simulink model "Practica3_ValeriaSinaiLaraRojas"  (R2025b)
settings: Solver=ode23t  StartTime=0.0  StopTime=10  RelTol=1e-3
libraries: fl_lib x22, nesl_utility x10
settings Model: Creator=Cecilia  LastModifiedBy=Cecilia

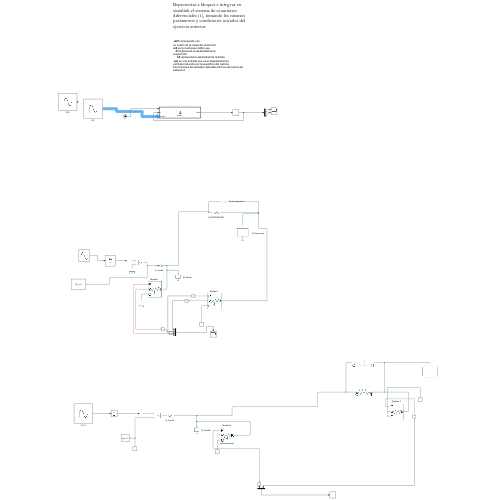
[thumbnail: Simulink's stored preview of the top-level diagram]
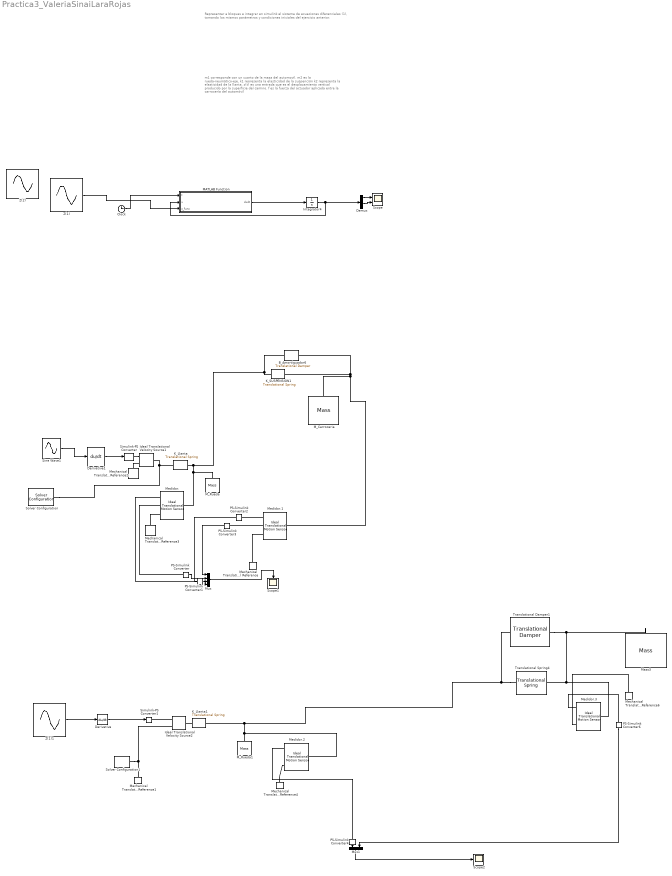
== system Practica3_ValeriaSinaiLaraRojas ==
  note: m1 corresponde con
      | un cuarto de la masa del automovil.
      | m2 es la rueda-neumático-eje,
      | k1 representa la elasticidad de la
      | suspención
      | k2 representa la elasticidad de la llanta.
      | z(t) es una entrada que es el desplazamiento
      | vertical producido por la superficie del camino.
      | f es la fuerza del actuador aplicada entre la carrocería del
      | automóvil
  note: Representar a bloques e integrar en simulink el sistema de ecuaciones diferenciales (1), tomando los mismos
      | parámetros y condiciones iniciales del ejercicio anterior.
  B_Amortiguador6 : fl_lib/Mechanical/Translational Elements/Translational Damper  D=1000 N*s/m  v_specify=off  v_priority=None  v=0 m/s  v_nominal_specify=off  v_nominal_value=1  v_nominal_unit=m/s  f_specify=off  f_priority=None  f=0 N  f_nominal_specify=off  f_nominal_value=1  f_nominal_unit=N
  Clock : Clock
  Demux : Demux
  Derivative : Derivative
  Derivative1 : Derivative
  Ideal Translational Velocity Source1 : fl_lib/Mechanical/Mechanical Sources/Ideal Translational Velocity Source
  Ideal Translational Velocity Source2 : fl_lib/Mechanical/Mechanical Sources/Ideal Translational Velocity Source
  Integrator4 : Integrator  InitialCondition=[0; 0; 0; 0]
  K_Llanta : fl_lib/Mechanical/Translational Elements/Translational Spring  spr_rate=19000 N/m  v_specify=off  v_priority=None  v=0 m/s  v_nominal_specify=off  v_nominal_value=1  v_nominal_unit=m/s  f_specify=off  f_priority=None  f=0 N  f_nominal_specify=off  f_nominal_value=1  f_nominal_unit=N  x_specify=off  x_priority=High  x=0 m  x_nominal_specify=off  x_nominal_value=1  x_nominal_unit=m
  K_Llanta1 : fl_lib/Mechanical/Translational Elements/Translational Spring  spr_rate=19000 N/m  v_specify=off  v_priority=None  v=0 m/s  v_nominal_specify=off  v_nominal_value=1  v_nominal_unit=m/s  f_specify=off  f_priority=None  f=0 N  f_nominal_specify=off  f_nominal_value=1  f_nominal_unit=N  x_specify=off  x_priority=High  x=0 m  x_nominal_specify=off  x_nominal_value=1  x_nominal_unit=m
  K_SUSPENSION1 : fl_lib/Mechanical/Translational Elements/Translational Spring  spr_rate=16182 N/m  v_specify=off  v_priority=None  v=0 m/s  v_nominal_specify=off  v_nominal_value=1  v_nominal_unit=m/s  f_specify=off  f_priority=None  f=0 N  f_nominal_specify=off  f_nominal_value=1  f_nominal_unit=N  x_specify=off  x_priority=High  x=0 m  x_nominal_specify=off  x_nominal_value=1  x_nominal_unit=m
  MATLAB Function : MATLAB Function  TreatAsAtomicUnit=on
  M_Carroceria : fl_lib/Mechanical/Translational Elements/Mass  mass=290 kg  num_ports=foundation.enum.numPorts2.one  v_specify=on  v_priority=High  v=1 m/s  v_nominal_specify=on  v_nominal_value=1  v_nominal_unit=m/s  f_specify=off  f_priority=None  f=0 N  f_nominal_specify=off  f_nominal_value=1  f_nominal_unit=N
  M_Rueda : fl_lib/Mechanical/Translational Elements/Mass  mass=59 kg  num_ports=foundation.enum.numPorts2.one  v_specify=off  v_priority=High  v=0 m/s  v_nominal_specify=off  v_nominal_value=1  v_nominal_unit=m/s  f_specify=off  f_priority=None  f=0 N  f_nominal_specify=off  f_nominal_value=1  f_nominal_unit=N
  M_Rueda1 : fl_lib/Mechanical/Translational Elements/Mass  mass=59 kg  num_ports=foundation.enum.numPorts2.one  v_specify=off  v_priority=High  v=0 m/s  v_nominal_specify=off  v_nominal_value=1  v_nominal_unit=m/s  f_specify=off  f_priority=None  f=0 N  f_nominal_specify=off  f_nominal_value=1  f_nominal_unit=N
  Mass3 : fl_lib/Mechanical/Translational Elements/Mass  mass=290 kg  num_ports=foundation.enum.numPorts2.one  v_specify=on  v_priority=High  v=0 m/s  v_nominal_specify=on  v_nominal_value=1  v_nominal_unit=m/s  f_specify=off  f_priority=None  f=0 N  f_nominal_specify=off  f_nominal_value=1  f_nominal_unit=N
  Mechanical Translational Reference{,1..4,6} (6 alike) : fl_lib/Mechanical/Translational Elements/Mechanical Translational Reference
  Medidor.{,1..3} (4 alike) : fl_lib/Mechanical/Mechanical Sensors/Ideal Translational Motion Sensor  reference=foundation.enum.MeasurementReference.difference  acceleration_port=false  velocity_port=true  position_port=true  offset=0 m
  Mux : Mux
  Mux1 : Mux  Inputs=2
  PS-Simulink Converter{,1..4,6} (6 alike) : nesl_utility/PS-Simulink Converter  PhysicalDomain=network_engine_domain  SubClassName=ps_output  LeftPortType=input  RightPortType=output  PseudoPeriodic=off  Frequencies=[]  VectorFormat=inherit  Unit=inherit  AffineConversion=off
  Scope : Scope  NumInputPorts=2
      settings: ActiveDisplayYMinimum=-0.061836360748085892  ActiveDisplayYMaximum=0.068675886807107581
  Scope1 : Scope
      settings: ActiveDisplayYMinimum=-1.0241021314644039  ActiveDisplayYMaximum=1.2249002368293782
  Scope2 : Scope
      settings: ActiveDisplayYMinimum=-0.12212269763999509  ActiveDisplayYMaximum=0.10067538321812189  DataLoggingVariableName=ScopeData2
  Simulink-PS Converter : nesl_utility/Simulink-PS Converter  PhysicalDomain=network_engine_domain  SubClassName=ps_input  LeftPortType=input  RightPortType=output  PseudoPeriodic=off  Frequencies=[]  NoiseDistribution=none  NoiseParameters=[]  Unit=1  AffineConversion=off  FilteringAndDerivatives=provide  SimscapeFilterOrder=1  InputFilterTimeConstant=0.001  UdotUserProvided=0
  Simulink-PS Converter1 : nesl_utility/Simulink-PS Converter  PhysicalDomain=network_engine_domain  SubClassName=ps_input  LeftPortType=input  RightPortType=output  PseudoPeriodic=off  Frequencies=[]  NoiseDistribution=none  NoiseParameters=[]  Unit=1  AffineConversion=off  FilteringAndDerivatives=provide  SimscapeFilterOrder=1  InputFilterTimeConstant=0.001  UdotUserProvided=0
  Sine Wave1 : Sin  Amplitude=0.05  Frequency=20*pi  SampleTime=0
  Solver Configuration : nesl_utility/Solver Configuration  PhysicalDomain=network_engine_domain  SubClassName=solver  LeftPortType=input  RightPortType=generic  Tones=[]  Harmonics=[]  SimulateNoise=off  Profile=off  UseLocalSampling=off  EnableSwitchedLinearOptims=on  FrequencyDomain=off  UseCCode=off  RelTol=0.001  AbsTol=0.001  MinStep=1e-09  ToWorkspace=off  RevertToSquareIcSolve=off  NumHomotopyIterations=100  PhasorMode=off  PhasorModeNumHarmonics=1  ConsistencySolver=NEWTON_XTOL_AFTER_FTOL  IndexReductionMethod=DerivativeReplacement  DoDC=off  ResidualTolerance=1e-09  ConsistencyTolSource=GLOBAL  ConsistencyAbsTol=0.001  ConsistencyRelTol=0.001  ConsistencyTolFactor=0.001  UseLocalSolver=off  LocalSolverChoice=NE_BACKWARD_EULER_ADVANCER  ResolveIndetEquations=on  FunctionEvalNumThread=1  LocalSolverSampleTime=0.001  DoFixedCost=off  MaxNonlinIter=3  MaxModeIter=2  ComputeImpulses=off  ImpulseIterations=2  LinearAlgebra=auto  LinearAlgebraNumThread=0  EquationFormulation=NE_TIME_EF  DelaysMemoryBudget=1024  AutomaticFiltering=on  FilteringTimeConstant=0.001  PartitionStorageMethod=AS_NEEDED  PartitionMemoryBudget=1024  PartitionMethod=ROBUST  MultibodyUseLocalSolver=off  MultibodyLocalSolverChoice=ODE1  MultibodyLocalSolverSampleTime=0.001
  Solver Configuration1 : nesl_utility/Solver Configuration  PhysicalDomain=network_engine_domain  SubClassName=solver  LeftPortType=input  RightPortType=generic  Tones=[]  Harmonics=[]  SimulateNoise=off  Profile=off  UseLocalSampling=off  EnableSwitchedLinearOptims=on  FrequencyDomain=off  UseCCode=off  RelTol=0.001  AbsTol=0.001  MinStep=1e-09  ToWorkspace=off  RevertToSquareIcSolve=off  NumHomotopyIterations=100  PhasorMode=off  PhasorModeNumHarmonics=1  ConsistencySolver=NEWTON_XTOL_AFTER_FTOL  IndexReductionMethod=DerivativeReplacement  DoDC=off  ResidualTolerance=1e-09  ConsistencyTolSource=GLOBAL  ConsistencyAbsTol=0.001  ConsistencyRelTol=0.001  ConsistencyTolFactor=0.001  UseLocalSolver=off  LocalSolverChoice=NE_BACKWARD_EULER_ADVANCER  ResolveIndetEquations=on  FunctionEvalNumThread=1  LocalSolverSampleTime=0.001  DoFixedCost=off  MaxNonlinIter=3  MaxModeIter=2  ComputeImpulses=off  ImpulseIterations=2  LinearAlgebra=auto  LinearAlgebraNumThread=0  EquationFormulation=NE_TIME_EF  DelaysMemoryBudget=1024  AutomaticFiltering=on  FilteringTimeConstant=0.001  PartitionStorageMethod=AS_NEEDED  PartitionMemoryBudget=1024  PartitionMethod=ROBUST  MultibodyUseLocalSolver=off  MultibodyLocalSolverChoice=ODE1  MultibodyLocalSolverSampleTime=0.001
  Translational Damper1 : fl_lib/Mechanical/Translational Elements/Translational Damper  D=1000 N*s/m  v_specify=off  v_priority=None  v=0 m/s  v_nominal_specify=off  v_nominal_value=1  v_nominal_unit=m/s  f_specify=on  f_priority=None  f=0 N  f_nominal_specify=off  f_nominal_value=0  f_nominal_unit=N
  Translational Spring4 : fl_lib/Mechanical/Translational Elements/Translational Spring  spr_rate=16182 N/m  v_specify=off  v_priority=None  v=0 m/s  v_nominal_specify=off  v_nominal_value=1  v_nominal_unit=m/s  f_specify=on  f_priority=None  f=0 N  f_nominal_specify=off  f_nominal_value=1  f_nominal_unit=N  x_specify=off  x_priority=High  x=0 m  x_nominal_specify=off  x_nominal_value=1  x_nominal_unit=m
  Z(1) : Sin  Amplitude=0.05  Frequency=0.5*pi  SampleTime=0
  Z(1)1 : Sin  Amplitude=0.05  Frequency=0.5*pi  SampleTime=0
  Z(2) : Sin  Amplitude=0.05  Frequency=62.8319  SampleTime=0
  wires:
  Clock/1 -> MATLAB Function/1(t)
  MATLAB Function/1(dxdt) -> Integrator4/1
  Integrator4/1 -> Demux/1, MATLAB Function/2(x)
  Z(1)/1 -> MATLAB Function/3(z_func)
  Demux/3 -> Scope/2
  Demux/1 -> Scope/1
  Derivative1/1 -> Simulink-PS Converter/1
  PS-Simulink Converter1/1 -> Mux/4
  PS-Simulink Converter3/1 -> Mux/1
  PS-Simulink Converter/1 -> Mux/2
  PS-Simulink Converter2/1 -> Mux/3
  Z(1)1/1 -> Derivative/1
  Derivative/1 -> Simulink-PS Converter1/1
  PS-Simulink Converter4/1 -> Mux1/1
  Mux1/1 -> Scope2/1
  PS-Simulink Converter6/1 -> Mux1/2
  Mux/1 -> Scope1/1
  Sine Wave1/1 -> Derivative1/1
  connections:
  Mechanical Translational Reference2/LConn1 -- Ideal Translational Velocity Source1/RConn2
  Simulink-PS Converter/RConn1 -- Ideal Translational Velocity Source1/RConn1
  K_Llanta/LConn1 -- Solver Configuration/RConn1 -- Ideal Translational Velocity Source1/LConn1
  Medidor./RConn1 -- Mechanical Translational Reference3/LConn1
  PS-Simulink Converter1/LConn1 -- Medidor./RConn3
  PS-Simulink Converter/LConn1 -- Medidor./RConn2
  Medidor.1/RConn1 -- Mechanical Translational Reference/LConn1
  Medidor.1/RConn3 -- PS-Simulink Converter2/LConn1
  Medidor.1/RConn2 -- PS-Simulink Converter3/LConn1
  M_Carroceria/LConn1 -- K_SUSPENSION1/RConn1 -- B_Amortiguador6/RConn1 -- Medidor.1/LConn1
  Medidor./LConn1 -- M_Rueda/LConn1 -- K_Llanta/RConn1 -- B_Amortiguador6/LConn1 -- K_SUSPENSION1/LConn1
  Ideal Translational Velocity Source2/RConn1 -- Simulink-PS Converter1/RConn1
  Mechanical Translational Reference1/LConn1 -- Solver Configuration1/RConn1 -- Ideal Translational Velocity Source2/RConn2
  K_Llanta1/LConn1 -- Ideal Translational Velocity Source2/LConn1
  Translational Spring4/RConn1 -- Medidor.2/LConn1 -- M_Rueda1/LConn1 -- K_Llanta1/RConn1 -- Translational Damper1/RConn1
  Mechanical Translational Reference4/LConn1 -- Medidor.2/RConn1
  Medidor.2/RConn3 -- PS-Simulink Converter4/LConn1
  Mass3/LConn1 -- Translational Damper1/LConn1 -- Medidor.3/LConn1 -- Translational Spring4/LConn1
  Mechanical Translational Reference6/LConn1 -- Medidor.3/RConn1
  PS-Simulink Converter6/LConn1 -- Medidor.3/RConn3

== matlab function Practica3_ValeriaSinaiLaraRojas/MATLAB Function ==
  data: t input; x input; dxdt output; z_func input


function dxdt = Carro(t, x, z_func)

    m1 = 290; b1 = 1000; m2 = 59; k1 = 16182; k2 = 19000; f = 0;
    
    x1 = x(1); v1 = x(2); x2 = x(3); v2 = x(4);
    
    z = z_func;
    
    dxdt = zeros(4,1);
    dxdt(1) = v1;
    dxdt(2) = (1/m1) * (-b1*v1 + b1*v2 - k1*x1 + k1*x2 + f);
    dxdt(3) = v2;
    dxdt(4) = (1/m2) * (b1*v1 - b1*v2 + k1*x1 - (k1+k2)*x2 - f + k2*z);
end
